simulink model "aero_guidance_targetwith315"  (R2026a)
settings: Solver=FixedStepAuto  StopTime=20  FixedStep=0.001  AbsTol=1e-6
PreLoadFcn:
  | aero_guid_dat
StopFcn:
  | aero_guid_plot
values from neighbouring files (symbols this model uses):
  d2r = pi/180    (= 0.0174532925199)    [aero_guid_plot.m]
  target_dt = 0.01    [rl_target_params.m]
undefined symbols (not defined in the file or in its folder): alpha_sch, alpha_vec, Beamwidth, Cm_alpha, Cm_el, Cm_q, Cx_alpha, Cz_alpha, Cz_el, d_ref, fin_max, fin_min, g, h_ini, K, K_r, Ka, Kg, Ki, Ks, l_acc, M_sch, Mach_vec, max_acc, max_gimbal, min_gimbal, omegaDotMax, omegaPhysMax, pos_tgt, q_ini, S_ref, Thrust, tors, v_ini, v_tgt, wgyro, wn_hom, x_ini
libraries: aerolibasang x3, simulink x2, aerolibanim x1, aerolibatmos2 x1, aerolibactuator x1, rllib x1
(part 2 of 2)

== matlab function aero_guidance_targetwith315/Target/Local Maneuver Policy/MATLAB Function ==
  settings: updateMethod=DISCRETE
  data: Mode input; TargetPos input; TargetHeading input; MissilePos input; TargetSpeed input; Vc input; GimbalAngle input; LookAngle input; Acquire input; omegaEvade output; t input; gimbalUsage output; trackingError output; attackPhase output
function [omegaEvade, gimbalUsage, ...
          trackingError, attackPhase] = ...
    gimbalAttackCommand( ...
        Mode, TargetPos, TargetHeading, ...
        MissilePos, TargetSpeed, Vc, ...
        GimbalAngle, LookAngle, Acquire, t)
%#codegen
%
% Rule-based target evasion policy
%
% Mode
%   2 : Predictive Evasive Maneuver
%   3 : Predictive Terminal Evasion
%
% 좌표계
%   Xdot = V*cos(psi)
%   Zdot = V*sin(psi)
%
% 출력
%   omegaEvade   : 타겟 회전율 명령 [rad/s]
%   gimbalUsage  : 짐벌 한계 사용률
%   trackingError: LookAngle - GimbalAngle [rad]
%   attackPhase
%       0 : 비회피
%       5 : Predictive Terminal Rule
%       6 : Predictive Evasive Rule

%% ============================================================
% Persistent state for simulation reset detection
% =============================================================

persistent initialized
persistent previousTime

if isempty(initialized)
    initialized = true;
    previousTime = t;
end

% 시뮬레이션이 다시 시작된 경우
if t < previousTime
    resetPredictiveEvasiveRule();
    resetPredictiveTerminalRule();
end

previousTime = t;

currentMode = uint8(Mode);

%% ============================================================
% Configuration
% =============================================================

gimbalLimit = 35.0*pi/180.0;

normalOmegaLimit   = 60.0*pi/180.0;
terminalOmegaLimit = 60.0*pi/180.0;

%% ============================================================
% Diagnostic metrics
% =============================================================

trackingError = wrapAngleLocal( ...
    LookAngle - GimbalAngle);

gimbalUsage = ...
    abs(GimbalAngle)/max(gimbalLimit,1.0e-6);

% 진단값이 과도하게 커지는 것만 방지
gimbalUsage = min(gimbalUsage,2.0);

omegaEvade = 0.0;
attackPhase = 0.0;

%% ============================================================
% Non-evasive modes
% =============================================================

if currentMode ~= uint8(2) && ...
   currentMode ~= uint8(3)

    return;
end

%% ============================================================
% Mode 3: Predictive Terminal Rule
% =============================================================

if currentMode == uint8(3)

    omegaEvade = predictiveTerminalRule( ...
        TargetPos, TargetHeading, ...
        MissilePos, TargetSpeed, Vc, ...
        terminalOmegaLimit, t);

    omegaEvade = min( ...
        max(omegaEvade,-terminalOmegaLimit), ...
        terminalOmegaLimit);

    attackPhase = 5.0;
    return;
end

%% ============================================================
% Mode 2: Predictive Evasive Rule
% =============================================================

omegaEvade = predictiveEvasiveRule( ...
    TargetPos, TargetHeading, ...
    MissilePos, TargetSpeed, Vc, ...
    GimbalAngle, LookAngle, Acquire, ...
    normalOmegaLimit, t);

omegaEvade = min( ...
    max(omegaEvade,-normalOmegaLimit), ...
    normalOmegaLimit);

attackPhase = 6.0;

end


%% ============================================================
% Mode 2: Predictive Evasive Rule
% =============================================================

function omegaEvasive = predictiveEvasiveRule( ...
    TargetPos, TargetHeading, ...
    MissilePos, TargetSpeed, Vc, ...
    GimbalAngle, LookAngle, Acquire, ...
    omegaLimit, t)
%#codegen
%
% 여러 회전율 후보를 짧은 시간 동안 예측한 뒤,
% 거리 확보와 LOS 변화에 유리한 후보를 선택한다.

persistent initialized
persistent previousMissilePos
persistent previousTime
persistent previousOmega
persistent selectedSign
persistent lastDirectionChangeTime

if isempty(initialized)
    initialized = true;

    previousMissilePos = MissilePos;
    previousTime = t;
    previousOmega = 0.0;

    selectedSign = 1.0;
    lastDirectionChangeTime = t;
end

%% 시뮬레이션 재시작 처리

if t < previousTime
    previousMissilePos = MissilePos;
    previousTime = t;
    previousOmega = 0.0;

    selectedSign = 1.0;
    lastDirectionChangeTime = t;
end

%% 미사일 속도 추정

measurementDt = t - previousTime;

if measurementDt > 1.0e-6

    missileVelocity = ...
        (MissilePos - previousMissilePos)/measurementDt;

else

    missileVelocity = [0.0; 0.0];
end

previousMissilePos = MissilePos;
previousTime = t;

%% 현재 상대 기하

currentRel = TargetPos - MissilePos;

currentRange = hypot( ...
    currentRel(1), ...
    currentRel(2));

currentLOS = atan2( ...
    currentRel(2), ...
    currentRel(1));

currentTrackingError = wrapAngleLocal( ...
    LookAngle - GimbalAngle);

acquired = Acquire > 0.5;

%% 위험도 계산

% R >= 3500 m이면 0
% R <= 900 m이면 1
rangeUrgency = ...
    (3500.0-currentRange)/(3500.0-900.0);

rangeUrgency = min( ...
    max(rangeUrgency,0.0), ...
    1.0);

% Vc <= 0이면 0
% Vc >= 500 m/s이면 1
closingUrgency = ...
    min(max(Vc/500.0,0.0),1.0);

urgency = max( ...
    rangeUrgency, ...
    closingUrgency);

%% 예측 시간

% 원거리에서는 긴 미래를 보고,
% 근거리에서는 짧고 빠르게 대응
predictionTime = ...
    0.70 - 0.30*urgency;

numberOfSteps = 12;

predictionDt = ...
    predictionTime/double(numberOfSteps);

%% 후보 회전율

candidateFractions = [
    -1.00;
    -0.70;
    -0.35;
     0.00;
     0.35;
     0.70;
     1.00
];

numberOfCandidates = 7;

%% 점수 가중치

finalRangeWeight = 4.0;
minRangeWeight   = 6.0;
losChangeWeight  = 1.4;
gimbalWeight     = 0.8;

effortWeight = 0.10;
changeWeight = 0.35;

bestScore = -1.0e12;
bestOmega = previousOmega;
bestSign = selectedSign;

%% ============================================================
% 후보 평가
% =============================================================

for candidateIndex = 1:numberOfCandidates

    candidateOmega = ...
        candidateFractions(candidateIndex) ...
        * abs(omegaLimit);

    predictedTargetPos = TargetPos;
    predictedTargetHeading = TargetHeading;
    predictedMissilePos = MissilePos;

    predictedMinRange = currentRange;

    %% 미래 궤적 예측

    for stepIndex = 1:numberOfSteps

        predictedTargetHeading = wrapAngleLocal( ...
            predictedTargetHeading ...
            + candidateOmega*predictionDt);

        predictedTargetVelocity = ...
            TargetSpeed * ...
            [cos(predictedTargetHeading);
             sin(predictedTargetHeading)];

        predictedTargetPos = ...
            predictedTargetPos ...
            + predictedTargetVelocity*predictionDt;

        predictedMissilePos = ...
            predictedMissilePos ...
            + missileVelocity*predictionDt;

        predictedRelStep = ...
            predictedTargetPos ...
            - predictedMissilePos;

        predictedRangeStep = hypot( ...
            predictedRelStep(1), ...
            predictedRelStep(2));

        predictedMinRange = min( ...
            predictedMinRange, ...
            predictedRangeStep);
    end

    %% 예측 종료 시 상대거리

    predictedRel = ...
        predictedTargetPos ...
        - predictedMissilePos;

    predictedFinalRange = hypot( ...
        predictedRel(1), ...
        predictedRel(2));

    %% 예측 LOS 변화

    predictedLOS = atan2( ...
        predictedRel(2), ...
        predictedRel(1));

    predictedLOSChange = abs( ...
        wrapAngleLocal( ...
            predictedLOS-currentLOS));

    %% 거리 점수

    finalRangeProgress = ...
        (predictedFinalRange-currentRange)/100.0;

    minRangeProgress = ...
        (predictedMinRange-currentRange)/100.0;

    %% 짐벌 부담 근사

    predictedGimbalStress = ...
        abs(currentTrackingError) ...
        + predictedLOSChange;

    %% 조종 비용

    normalizedEffort = ...
        candidateOmega ...
        /max(abs(omegaLimit),1.0e-6);

    normalizedChange = ...
        (candidateOmega-previousOmega) ...
        /max(abs(omegaLimit),1.0e-6);

    %% 기본 점수

    score = ...
          finalRangeWeight*finalRangeProgress ...
        + minRangeWeight*minRangeProgress ...
        + losChangeWeight ...
            *(predictedLOSChange/(20.0*pi/180.0)) ...
        + gimbalWeight*predictedGimbalStress ...
        - effortWeight*normalizedEffort^2 ...
        - changeWeight*normalizedChange^2;

    %% 미사일 쪽으로 접근하는 후보 강한 감점

    if predictedFinalRange < currentRange

        score = score ...
            - 6.0 ...
            *(currentRange-predictedFinalRange)/100.0;
    end

    if predictedMinRange < currentRange-30.0

        score = score ...
            - 8.0 ...
            *(currentRange-predictedMinRange)/100.0;
    end

    %% Lock이 끊긴 경우 거리 확보를 더 우선

    if ~acquired

        score = score ...
            + 4.0*finalRangeProgress ...
            + 5.0*minRangeProgress;
    end

    %% 가장 좋은 후보 선택

    if score > bestScore

        bestScore = score;
        bestOmega = candidateOmega;
        bestSign = signNonzero(candidateOmega);
    end
end

%% ============================================================
% 너무 빠른 좌우 반전 방지
% =============================================================

minimumDirectionHoldTime = ...
    0.30 - 0.08*urgency;

directionChanged = ...
    bestSign ~= selectedSign;

if directionChanged && ...
   abs(previousOmega) > 1.0*pi/180.0

    if (t-lastDirectionChangeTime) ...
            < minimumDirectionHoldTime

        % 최소 유지시간 전에는 기존 방향 유지
        bestOmega = selectedSign*abs(bestOmega);

    else

        selectedSign = bestSign;
        lastDirectionChangeTime = t;
    end
end

%% 직진 후보가 선택된 경우 sign 유지

if abs(bestOmega) < 1.0*pi/180.0
    bestSign = selectedSign;
end

%% ============================================================
% 명령 완화
% =============================================================

% 가까울수록 후보 명령을 더 빠르게 반영
commandResponse = ...
    0.50 + 0.35*urgency;

omegaEvasive = ...
      (1.0-commandResponse)*previousOmega ...
    + commandResponse*bestOmega;

omegaEvasive = min( ...
    max(omegaEvasive,-omegaLimit), ...
    omegaLimit);

previousOmega = omegaEvasive;

end


%% ============================================================
% Mode 3: Predictive Terminal Rule
% =============================================================

function omegaTerminal = predictiveTerminalRule( ...
    TargetPos, TargetHeading, ...
    MissilePos, TargetSpeed, Vc, ...
    omegaLimit, t)
%#codegen
%
% 근거리에서 좌·우 최대 선회 후보를 짧게 예측하고,
% 예상 분리거리가 더 큰 방향을 선택한다.

persistent initialized
persistent previousSelectedSign
persistent previousCommand
persistent lastSwitchTime
persistent previousTime

if isempty(initialized)
    initialized = true;

    previousSelectedSign = 1.0;
    previousCommand = 0.0;

    lastSwitchTime = t;
    previousTime = t;
end

%% 시뮬레이션 재시작 처리

if t < previousTime
    previousSelectedSign = 1.0;
    previousCommand = 0.0;

    lastSwitchTime = t;
end

previousTime = t;

%% 위험도

closingFactor = ...
    min(max(Vc/500.0,0.0),1.0);

omegaCandidate = ...
    (0.85 + 0.15*closingFactor) ...
    * abs(omegaLimit);

predictionTime = ...
    0.28 + 0.08*(1.0-closingFactor);

currentRel = ...
    TargetPos - MissilePos;

currentRange = hypot( ...
    currentRel(1), ...
    currentRel(2));

%% ============================================================
% 양의 선회 후보
% =============================================================

headingPlus = wrapAngleLocal( ...
    TargetHeading ...
    + omegaCandidate*predictionTime);

targetMovePlus = ...
    TargetSpeed*predictionTime * ...
    [cos(headingPlus);
     sin(headingPlus)];

predictedRelPlus = ...
    currentRel + targetMovePlus;

rangePlus = hypot( ...
    predictedRelPlus(1), ...
    predictedRelPlus(2));

%% ============================================================
% 음의 선회 후보
% =============================================================

headingMinus = wrapAngleLocal( ...
    TargetHeading ...
    - omegaCandidate*predictionTime);

targetMoveMinus = ...
    TargetSpeed*predictionTime * ...
    [cos(headingMinus);
     sin(headingMinus)];

predictedRelMinus = ...
    currentRel + targetMoveMinus;

rangeMinus = hypot( ...
    predictedRelMinus(1), ...
    predictedRelMinus(2));

%% 후보 차이

rangeAdvantage = ...
    rangePlus-rangeMinus;

switchThreshold = 8.0;

candidateSign = previousSelectedSign;

if rangeAdvantage > switchThreshold

    candidateSign = 1.0;

elseif rangeAdvantage < -switchThreshold

    candidateSign = -1.0;
end

%% 너무 잦은 좌우 전환 방지

minimumHoldTime = ...
    0.18 + 0.07*(1.0-closingFactor);

if candidateSign ~= previousSelectedSign

    if (t-lastSwitchTime) >= minimumHoldTime

        previousSelectedSign = candidateSign;
        lastSwitchTime = t;
    end
end

desiredCommand = ...
    previousSelectedSign*omegaCandidate;

%% 명령의 갑작스러운 점프 완화

commandResponse = ...
    0.80 + 0.15*closingFactor;

omegaTerminal = ...
      (1.0-commandResponse)*previousCommand ...
    + commandResponse*desiredCommand;

%% 분리거리가 감소 중이면 최대 명령에 가깝게 적용

if max(rangePlus,rangeMinus) < currentRange

    omegaTerminal = ...
        previousSelectedSign*abs(omegaLimit);
end

omegaTerminal = min( ...
    max(omegaTerminal,-omegaLimit), ...
    omegaLimit);

previousCommand = omegaTerminal;

end


%% ============================================================
% Reset helper for predictive evasive rule
% =============================================================

function resetPredictiveEvasiveRule()
%#codegen
%
% 코드 생성 호환을 위해 빈 헬퍼로 유지.
% 내부 persistent는 t 감소 조건에서 자체 초기화된다.

end


%% ============================================================
% Reset helper for predictive terminal rule
% =============================================================

function resetPredictiveTerminalRule()
%#codegen
%
% 코드 생성 호환을 위해 빈 헬퍼로 유지.
% 내부 persistent는 t 감소 조건에서 자체 초기화된다.

end


%% ============================================================
% Sign helper
% =============================================================

function outputSign = signNonzero(inputValue)
%#codegen

if inputValue > 0.0

    outputSign = 1.0;

elseif inputValue < 0.0

    outputSign = -1.0;

else

    outputSign = 1.0;
end

end


%% ============================================================
% Angle wrapping
% =============================================================

function angleWrapped = wrapAngleLocal(angleInput)
%#codegen

angleWrapped = atan2( ...
    sin(angleInput), ...
    cos(angleInput));

end

== matlab function aero_guidance_targetwith315/Target/MATLAB Function ==
  data: TargetPos input; omegaGoal output; TargetHeading input; goalDistance output; goalReached output; GoalPos input
function [omegaGoal, goalDistance, goalReached] = ...
    goalGuidance(TargetPos, TargetHeading, GoalPos)
%#codegen
%
% TargetPos     : [Xt; Zt] [m]
% TargetHeading : target heading [rad]
% GoalPos       : [Xgoal; Zgoal] [m]
%
% Target Dynamics:
% Xdot = V*cos(psi)
% Zdot = V*sin(psi)

GoalRadius = 100.0;   % 목표 도달 판정 반경 [m]

%% 목표까지 상대 위치
dx = GoalPos(1) - TargetPos(1);
dz = GoalPos(2) - TargetPos(2);

%% 목표까지 거리
goalDistance = hypot(dx, dz);

%% 목표 방향
% 현재 좌표계:
% Xdot = V*cos(psi)
% Zdot = V*sin(psi)
desiredHeading = atan2(dz, dx);

%% 목표 방향과 현재 Heading 차이
headingError = atan2( ...
    sin(desiredHeading - TargetHeading), ...
    cos(desiredHeading - TargetHeading));

%% 목표 추종 회전율
Kheading = 1.5;

% 최대 목표 추종 회전율: 30 deg/s
omegaGoalMax = 30.0*pi/180.0;

omegaGoal = Kheading * headingError;

%% 회전율 제한
omegaGoal = min( ...
    max(omegaGoal, -omegaGoalMax), ...
    omegaGoalMax);

%% 목표 도달 판정
goalReached = logical( ...
    goalDistance <= GoalRadius);

end

== matlab function aero_guidance_targetwith315/Target/MATLAB Function1 ==
  data: Mode input; omegaGoal input; omegaCmd output; omegaEvade input; goalReached input; UseRL_state input
function omegaCmd = commandMixer( ...
    Mode, omegaGoal, omegaEvade, goalReached, UseRL_state)
%#codegen

if logical(goalReached)
    omegaCmd = 0.0;
    return;
end

switch uint8(Mode)

    case uint8(0)
        goalWeight  = 1.00;
        evadeWeight = 0.00;

    case uint8(1)
        goalWeight  = 1.00;
        evadeWeight = 0.00;

    case uint8(2)

        if logical(UseRL_state)
            % 학습된 RL 행동을 그대로 적용
            goalWeight  = 0.00;
            evadeWeight = 1.00;
        else
            % 규칙 기반 회피에는 목표 추종을 일부 유지
            goalWeight  = 0.25;
            evadeWeight = 1.00;
        end

    case uint8(3)
        goalWeight  = 0.00;
        evadeWeight = 1.00;

    case uint8(4)
        goalWeight  = 1.00;
        evadeWeight = 0.00;

    case uint8(5)
        goalWeight  = 0.00;
        evadeWeight = 0.00;

    otherwise
        goalWeight  = 0.00;
        evadeWeight = 0.00;
end

omegaCmd = ...
    goalWeight*omegaGoal ...
    + evadeWeight*omegaEvade;

omegaLimit = 160*pi/180;

omegaCmd = min( ...
    max(omegaCmd,-omegaLimit), ...
    omegaLimit);

end

== matlab function aero_guidance_targetwith315/Target/Observation Builder ==
  data: dX input; dZ input; observation output; R input; Vc input; TargetHeading input; UseRL_state input; TargetPos input; GoalPos input
function observation = buildObservation( ...
    dX, dZ, R, Vc, ...
    TargetHeading, UseRL_state, ...
    TargetPos, GoalPos)
%#codegen
%
% Agent315 학습 환경과 동일한 9×1 Observation
%
% dX = TargetX - MissileX
% dZ = TargetZ - MissileZ
% Vc = closing velocity, 접근 중 양수

R_scale = 5000.0;
V_scale = 1000.0;

% 학습 모델은 Discrete Derivative로 dR/dt를 사용함.
% 현재 Demo에서 Vc가 접근 중 양수라면 dR/dt = -Vc
rangeRateRaw = -Vc;

goalDX = GoalPos(1) - TargetPos(1);
goalDZ = GoalPos(2) - TargetPos(2);

observation = zeros(9,1);

observation(1) = R  / R_scale;
observation(2) = dX / R_scale;
observation(3) = dZ / R_scale;
observation(4) = rangeRateRaw / V_scale;

observation(5) = sin(TargetHeading);
observation(6) = cos(TargetHeading);

% 학습 환경의 use_RL 신호
observation(7) = double(UseRL_state);

observation(8) = goalDX / R_scale;
observation(9) = goalDZ / R_scale;

end

== matlab function aero_guidance_targetwith315/Target/MATLAB Function2 ==
  data: action input; omegaRL output; Mode input; omegaPhysMax input
function omegaRL = actionMapper(action, Mode, omegaPhysMax)
%#codegen
%
% action       : RL Agent output [-1,1]
% Mode         : Stateflow flight mode
% omegaPhysMax : 학습 당시 최대 회전율 [rad/s]

action = min(max(action,-1.0),1.0);

switch uint8(Mode)

    case uint8(2)
        % 일반 회피 계열에서만 RL 명령을 계산
        % 실제로 이 명령을 사용할지는 UseRL_state가 결정
        omegaRL = action * omegaPhysMax;

    case uint8(3)
        % 터미널 상태는 현재 규칙 기반으로 유지
        omegaRL = 0.0;

    otherwise
        omegaRL = 0.0;
end

end

== matlab function aero_guidance_targetwith315/Target/Episode Logic ==
  data: R input; hit output; goalReached input; t input; timeout output; isDone output
function [hit, timeout, isDone] = ...
    episodeLogic(R, goalReached, t)
%#codegen

% 현재 모델의 실제 요격 판정 반경과 맞춰서 수정
hitRadius = 20.0;       % [m]

% 최대 에피소드 시간
episodeTime = 20.0;     % [s]

hit = (R <= hitRadius);
timeout = (t >= episodeTime);

isDone = ...
    hit || goalReached || timeout;

end

== matlab function aero_guidance_targetwith315/Target/MATLAB Function3 ==
  settings: updateMethod=DISCRETE  sampleTime=target_dt
  data: R input; reward output; goalDistance input; actionPrev input; goalReached input; hit input; timeout input; t input
function reward = targetReward( ...
    R, goalDistance, actionPrev, ...
    goalReached, hit, timeout, t)
%#codegen
%
% R            : 현재 미사일-타겟 거리 [m]
% goalDistance : 현재 목표까지 거리 [m]
% actionPrev   : 직전 Agent 행동, 스칼라 [-1, 1]
% goalReached  : 목표 도달 여부
% hit          : 요격 여부
% timeout      : 제한시간 초과 여부
% t            : 현재 시뮬레이션 시간 [s]
%
% reward       : 스칼라 double

%% 이전 Agent step의 상태 저장
persistent initialized
persistent prevR
persistent prevGoalDistance
persistent prevTime

if isempty(initialized)
    initialized = false;
    prevR = 0.0;
    prevGoalDistance = 0.0;
    prevTime = -1.0;
end

%% 출력 형식 명시
reward = 0.0;

%% 새로운 에피소드인지 판단
%
% 첫 실행이거나,
% Fast Restart 등으로 시간이 다시 0으로 돌아간 경우 초기화
newEpisode = ...
    (~initialized) || ...
    (t < prevTime) || ...
    (t <= 1.0e-12);

if newEpisode
    prevR = R;
    prevGoalDistance = goalDistance;
    prevTime = t;
    initialized = true;

    reward = 0.0;
    return;
end

%% 직전 Agent step 대비 진행량

% 미사일과 거리가 증가하면 양수
separationProgress = ...
    (R - prevR) / 100.0;

% 목표까지 거리가 감소하면 양수
goalProgress = ...
    (prevGoalDistance - goalDistance) / 100.0;

% 순간적인 비정상 값이 보상을 지나치게 크게 만들지 않도록 제한
separationProgress = min( ...
    max(separationProgress, -5.0), ...
    5.0);

goalProgress = min( ...
    max(goalProgress, -5.0), ...
    5.0);

%% 일반 보상

% 1. 미사일과 멀어지기
separationReward = ...
    0.30 * separationProgress;

% 2. 목표에 가까워지기
goalReward = ...
    0.70 * goalProgress;

% 3. 과도한 회피 명령 억제
actionPenalty = ...
    0.02 * actionPrev * actionPrev;

% 4. 불필요하게 오래 비행하는 것 억제
timePenalty = 0.002;

reward = ...
      separationReward ...
    + goalReward ...
    - actionPenalty ...
    - timePenalty;

%% 종료 보상
% 요격과 목표 도달이 동시에 검출되면 요격 실패를 우선 적용

if logical(hit)
    reward = -500.0;

elseif logical(goalReached)
    reward = 500.0;

elseif logical(timeout)
    reward = -50.0;
end

%% 다음 Agent step을 위해 현재 상태 저장

prevR = R;
prevGoalDistance = goalDistance;
prevTime = t;

end

== stateflow chart aero_guidance_targetwith315/Guidance/Guidance Processor (Updated @100Hz) ==
  settings: updateMethod=DISCRETE  sampleTime=0.01
  state Guidance [parallel]
    settings: executionOrder=1
    state Target_Search
      en: Mode=1;Sigma_d=0;incr=-100;Acquire_time=t;
      du: Sigma_d=Sigma_d+0.01*incr;
      Target_Search -> Target_Search [order 1] : [Sigma_d>30||Sigma_d<-30]  / incr=-incr;
    state Target_Lock
      en:Mode=2;Acquire_time=t;
    state Abort
      en:Detonate=1;
    state Radar_Guided
      en:Mode=3;
      ex:az_fix=az_dem;
    state Blind_Range
      en:Mode=4;
    (default) -> Target_Search : {az_fix=-9.81;}
    Radar_Guided -> Target_Search [order 1] : [Acquire==0]
    Target_Search -> Abort [order 2] : [t-Acquire_time>10]
        | / send(Timeout, Fuze);
    Target_Search -> Target_Lock [order 1] : [Acquire==1]
    Target_Lock -> Radar_Guided : [t-Acquire_time>0.2]
    Radar_Guided -> Blind_Range [order 2] : [Range<200]
  state Fuze [parallel]
    settings: executionOrder=2
    state Armed
      en:Fuze=1;
    state Inert
      en:Fuze = 0;
    Inert -> Armed [order 2] : [in(Guidance.Radar_Guided)&&Range<1000]
    (default) -> Inert
    Inert -> Armed [order 1] : Timeout
    Armed -> Inert : enter(Guidance.Target_Search)
  data: Range input double; Detonate output boolean; Fuze output boolean; Sigma_d output double; Mode output uint8; Acquire input boolean; Acquire_time local double; incr local double; az_dem input double; az_fix output double =-9.81
  data Sigma_d settings: description=Demanded Seeker Look Angle
  data Acquire settings: description=Seeker Acquisition Flag
  data incr settings: description=Seeker Search Rate
  events: Timeout local EITHER_EDGE_EVENT
